simulink subsystem "tiltAngleComplementaryFilter"  (R2024a)
settings: Solver=VariableStepAuto  StartTime=0.0  StopTime=10.0  RelTol=1e-3
undefined symbols (not defined in the file or in its folder): alpha, angleEstRate, controlRate
settings Model: Creator=Peter  LastModifiedBy=Peter

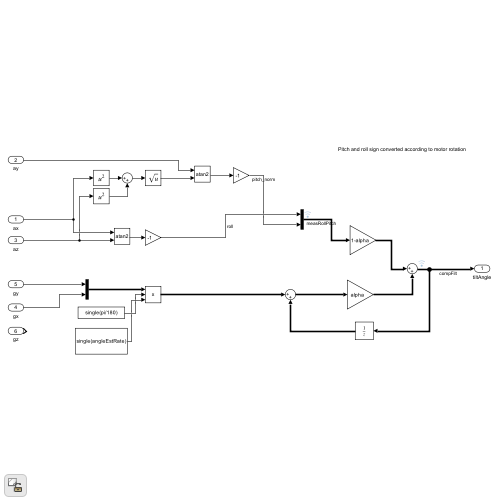
[thumbnail: Simulink's stored preview of the top-level diagram]
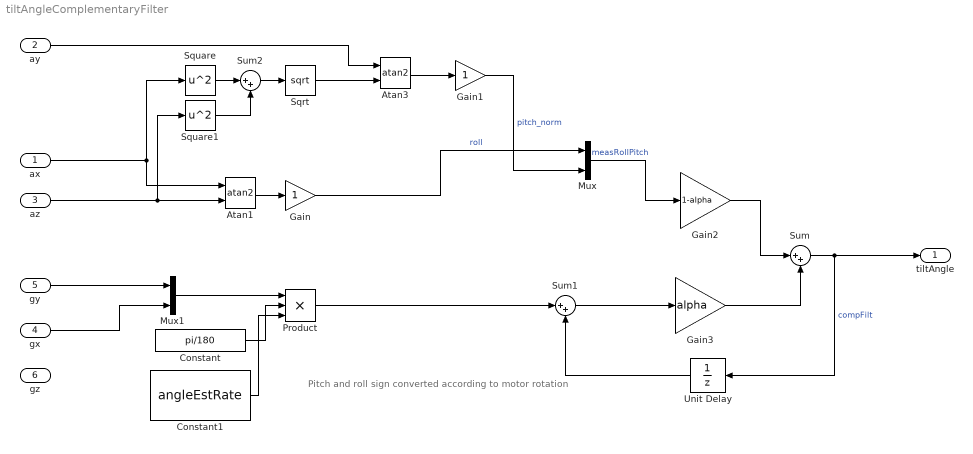
== system tiltAngleComplementaryFilter ==
  note: Pitch and roll sign converted according to motor rotation
  ax : Inport
  ay : Inport  Port=2
  az : Inport  Port=3
  gx : Inport  Port=4
  gy : Inport  Port=5
  gz : Inport  Port=6
  Atan1 : Trigonometry  Operator=atan2
  Atan3 : Trigonometry  Operator=atan2
  Constant : Constant  Value=pi/180  OutDataTypeStr=single
  Constant1 : Constant  Value=angleEstRate  OutDataTypeStr=single
  Gain : Gain
  Gain1 : Gain  OutDataTypeStr=single
  Gain2 : Gain  Gain=1-alpha  OutDataTypeStr=single
  Gain3 : Gain  Gain=alpha  OutDataTypeStr=single
  Mux : Mux  Inputs=2
  Mux1 : Mux  Inputs=2
  Product : Product  Inputs=3
  Sqrt : Sqrt
  Square : Math  Operator=square
  Square1 : Math  Operator=square
  Sum : Sum  Inputs=|++
  Sum1 : Sum  Inputs=|++
  Sum2 : Sum  Inputs=|++
  Unit Delay : UnitDelay  SampleTime=controlRate  HasFrameUpgradeWarning=on
  tiltAngle : Outport
  wires:
  ay/1 -> Atan3/1
  Sum/1 -> tiltAngle/1, Unit Delay/1  "compFilt"
  ax/1 -> Atan1/1, Square/1
  Atan1/1 -> Gain/1
  Gain/1 -> Mux/1  "roll"
  Mux/1 -> Gain2/1  "measRollPitch"
  gy/1 -> Mux1/1
  gx/1 -> Mux1/2
  Mux1/1 -> Product/1
  Constant/1 -> Product/2
  Product/1 -> Sum1/1
  Gain2/1 -> Sum/1
  Gain3/1 -> Sum/2
  Unit Delay/1 -> Sum1/2
  Sum1/1 -> Gain3/1
  Square/1 -> Sum2/1
  Square1/1 -> Sum2/2
  Sum2/1 -> Sqrt/1
  Sqrt/1 -> Atan3/2
  Atan3/1 -> Gain1/1
  Constant1/1 -> Product/3
  az/1 -> Atan1/2, Square1/1
  Gain1/1 -> Mux/2  "pitch_norm"
